simulink model "bikecar"  (R2016a)
settings: Solver=ode45  StartTime=0.0  StopTime=t_final  MaxStep=maxstep  RelTol=1e-3
values from neighbouring files (symbols this model uses):
  a = [(-2/tau - 1/tau_0) 1/tau 1/tau; 1/tau -2/tau 1/tau; 1/tau 1/tau -2/tau]    [MAE_272A_HW2_Q1a.m]    (also in Vehicle_Dynamic_main.m = 0.624; Vehicle_Dynamic_main_V0.m = 0.624; Vehicle_Dynamic_main_V01.m = 0.624; Vehicle_Dynamic_main_V0605.m = 0.624)
  b = [1/A 0; 0 1/A; 0 0]    [MAE_272A_HW2_Q1a.m]    (also in Vehicle_Dynamic_main.m = 0.624; Vehicle_Dynamic_main_V0.m = 0.624; Vehicle_Dynamic_main_V01.m = 0.624; Vehicle_Dynamic_main_V0605.m = 0.624)
  Cf = 5e4    (= 50000)    [master.m]
  Cr = Ku*abyb*Cf    (= 30000)    [master.m]
  inits = zeros(5,1)    [master.m]
  Jy = 0.4*m*a*b    (= 864)    [master.m]    (also in simulation_1.m = 4250)
  m = m_total*weight_front    (= 118.8)    [Wegiht_Transfer_Calculator.m]    (also in master.m = 1600; simulation_1.m = 1800)
  strMag = 0.95    [master.m]
  tauS = 1/2/pi/2    (= 0.0795774715459)    [master.m]
  u0 = 65*8.94/20    (= 29.055)    [master.m]    (also in simulation_1.m = 27.7777777778)
settings Model: Creator=eigenvalue  LastModifiedBy=Lin
settings DataIOCC: LimitDataPoints=on  SaveFormat=Array  SaveOutput=off  SignalLogging=off  DSMLogging=off  SaveTime=off
settings DebuggingCC: AllowSymbolicDim=off
settings HardwareCC: ProdBitPerPointer=32  ProdLargestAtomicFloat=None  ProdIntDivRoundTo=Undefined  ProdEndianess=Unspecified  ProdWordSize=32  ProdHWDeviceType=32-bit Generic
settings ModelReferenceCC: PropagateSignalLabelsOutOfModel=off
settings ConfigComp: CovModelRefEnable=Off

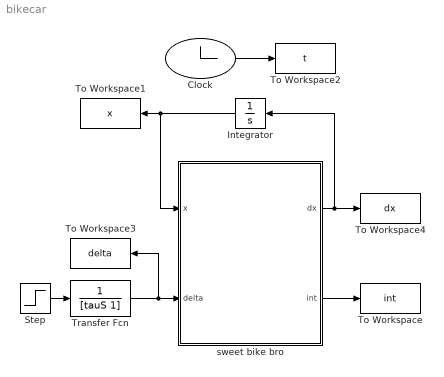
== system bikecar ==
  Clock : Clock
  Integrator : Integrator  InitialCondition=inits
  Step : Step  After=strMag*pi/180  SampleTime=0
  To Workspace : ToWorkspace  VariableName=int  SampleTime=-1
  To Workspace1 : ToWorkspace  VariableName=x  SampleTime=-1
  To Workspace2 : ToWorkspace  VariableName=t  SampleTime=-1
  To Workspace3 : ToWorkspace  VariableName=delta  SampleTime=-1
  To Workspace4 : ToWorkspace  VariableName=dx  SampleTime=-1
  Transfer Fcn : TransferFcn  Denominator=[tauS 1]
  sweet bike bro : MATLAB Function  TreatAsAtomicUnit=on
  wires:
  sweet bike bro/1(dx) -> Integrator/1, To Workspace4/1
  Integrator/1 -> To Workspace1/1, sweet bike bro/1(x)
  sweet bike bro/2(int) -> To Workspace/1
  Clock/1 -> To Workspace2/1
  Step/1 -> Transfer Fcn/1
  Transfer Fcn/1 -> To Workspace3/1, sweet bike bro/2(delta)

== matlab function bikecar/sweet bike bro ==
  data: x input; dx output; delta input; m parameter; Jy parameter; Cf parameter; Cr parameter; a parameter; b parameter; int output; u0 parameter
function [dx, int] = bike(x,delta, ...
    m,Jy,Cf,Cr,a,b,u0)
%#codegen
v = x(1);
wy = x(2);
psi = x(3);
dX = u0*cos(psi) - v*sin(psi);
dY = u0*sin(psi) + v*cos(psi);

alphaF = delta - v/u0 - a*wy/u0;
alphaR = -v/u0 + b*wy/u0;
FyF = Cf*alphaF; FyR = Cr*alphaR;
dv = 1/m*(FyF + FyR) - u0*wy;
dwy = 1/Jy*(a*FyF - b*FyR);
dpsi = wy;
lateracc = (FyF+FyR)/m/9.81;

dx = [dv; dwy; dpsi; dX; dY];
int = [alphaF; alphaR; lateracc];
